simulink model "Sim_localization_template"  (R2024b)
settings: Solver=VariableStepAuto  StartTime=0.0  StopTime=80  MaxStep=0.001  RelTol=1e-3
undefined symbols (not defined in the file or in its folder): D, d, d_actual, P_INIT_EKF, PHI_INIT, prob_gps_loss, Q_INIT, Q_INIT_LOC, r, R_2, R_3, R_4, R_5, r_actual, T_s, Ta, Tc, Z_INIT_EKF
settings Model: Creator=alberto  LastModifiedBy=Riccardo
settings RTWCC: GPUComputeCapability=3.5

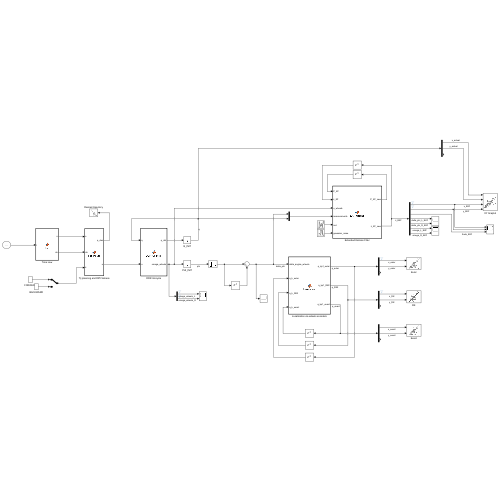
[thumbnail: Simulink's stored preview of the top-level diagram]
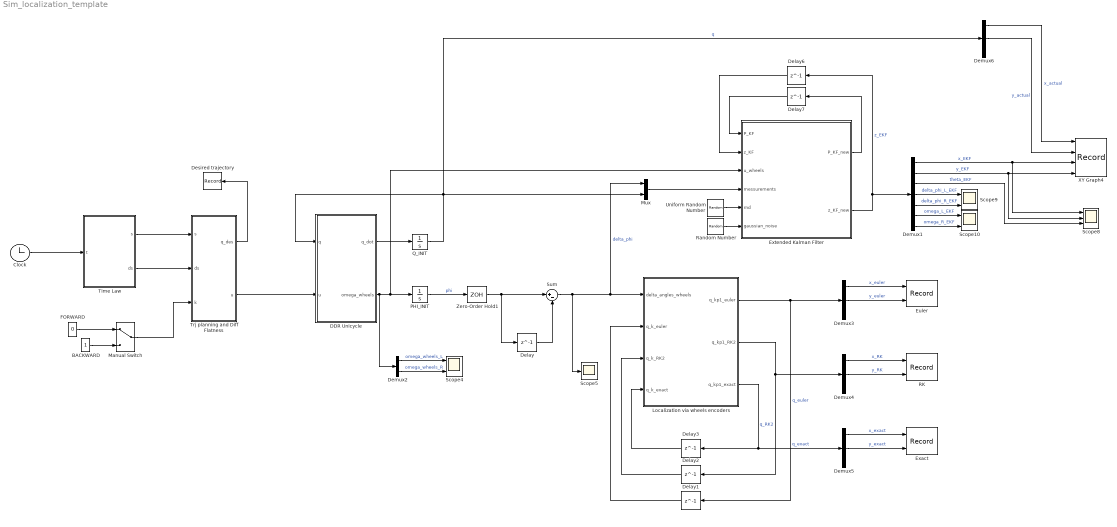
== system Sim_localization_template ==
  BACKWARD : Constant
  Clock : Clock
  DDR Unicycle : MATLAB Function  TreatAsAtomicUnit=on
  Delay : Delay  DelayLength=1  InitialCondition=[0;0]  SampleTime=T_s
  Delay1 : Delay  DelayLength=1  InitialCondition=Q_INIT_LOC
  Delay2 : Delay  DelayLength=1  InitialCondition=Q_INIT_LOC
  Delay3 : Delay  DelayLength=1  InitialCondition=Q_INIT_LOC
  Delay6 : Delay  DelayLength=1  InitialCondition=Z_INIT_EKF  SampleTime=T_s
  Delay7 : Delay  DelayLength=1  InitialCondition=P_INIT_EKF  SampleTime=T_s
  Demux1 : Demux  Outputs=7
  Demux2 : Demux  Outputs=2
  Demux{3..6} (4 alike) : Demux  Outputs=3
  Desired trajectory : Record  FileSettingsInternal="{\"entries\":[{\"content\":{\"excelSettings\":{\"content\":{},\"type\":\"Streamout.ExcelSettings\"}},\"type\":\"Streamout.FileSettingStorage\",\"uuid\":\"\"}],\"packageUris\":[\"http:\\/\\/schema.mathworks.com\\/mf0\\/streamout_blocks\\/R2020a\"],\"version\":\"1.0\"}"  Layout=[1 1]  SignalsInternal="{\"entries\":[{\"content\":{\"signals\":[{\"content\":{\"blockPath\":[],\"dimensions\":[3,1],\"domain\":\"\",\"hasChildren\":true,\"lineColor\":\"#0072bd\",\"lineWidth\":2,\"port\":1,\"sid\":[\"\"],\"signalID\":1,\"signalName\":\"Trj planning and Diff Flatness:1\"},\"type\":\"RecordBlkView.Signal\",\"uuid\":\"\"},{\"content\":{\"blockPath\":[],\"channel\":[1,1],\"dimensions\":[3,1],\"domain\":\"\",\"lineColor\":\"#b746ff\",\"lineWidth\":2,\"parentID\":1,\"plots\":[ 1 ],\"port\":1,\"sid\":[\"\"],\"signalID\":2,\"signalName\":\"Trj planning and Diff Flatness:1\"},\"type\":\"RecordBlkView.Signal\",\"uuid\":\"\"},{\"content\":{\"blockPath\":[],\"channel\":[2,1],\"dimensions\":[3,1],\"domain\":\"\",\"lineColor\":\"#64d413\",\"lineWidth\":2,\"parentID\":1,\"plots\":[ 1 ],\"port\":1,\"sid\":[\"\"],\"signalID\":3,\"signalName\":\"Trj planning and Diff Flatness:1\"},\"type\":\"RecordBlkView.Signal\",\"uuid\":\"\"},{\"content\":{\"blockPath\":[],\"channel\":[3,1],\"dimensions\":[3,1],\"domain\":\"\",\"lineColor\":\"#ff13a6\",\"lineWidth\":2,\"parentID\":1,\"port\":1,\"sid\":[\"\"],\"signalID\":4,\"signalName\":\"Trj planning and Diff Flatness:1\"},\"type\":\"RecordBlkView.Signal\",\"uuid\":\"\"}]},\"type\":\"RecordBlkView.InputSignals\",\"uuid\":\"\"}],\"packageUris\":[\"http:\\/\\/schema.mathworks.com\\/mf0\\/streamout_blocks\\/R2020a\"],\"version\":\"1.0\"}"  VisualizationBindings="{\"xyplotplugin\":{\"info\":[{\"series\":[{\"bindingParametersList\":[{\"parameter\":\"X-Axis\",\"signalID\":2,\"signalName\":\"Trj planning and Diff Flatness:1(1,1)\"},{\"parameter\":\"Y-Axis\",\"signalID\":3,\"signalName\":\"Trj planning and Diff Flatness:1(2,1)\"}],\"seriesID\":0}],\"subplotID\":1}]}}"  CompatibilityTag=XY
  Euler : Record  FileSettingsInternal="{\"entries\":[{\"content\":{\"excelSettings\":{\"content\":{},\"type\":\"Streamout.ExcelSettings\"}},\"type\":\"Streamout.FileSettingStorage\",\"uuid\":\"\"}],\"packageUris\":[\"http:\\/\\/schema.mathworks.com\\/mf0\\/streamout_blocks\\/R2020a\"],\"version\":\"1.0\"}"  Layout=[1 1]  SignalsInternal="{\"entries\":[{\"content\":{\"signals\":[{\"content\":{\"blockPath\":[],\"dimensions\":[1,1],\"domain\":\"\",\"lineColor\":\"#edb120\",\"lineWidth\":2,\"plots\":[ 1 ],\"port\":1,\"sid\":[\"\"],\"signalID\":1,\"signalName\":\"x_euler\"},\"type\":\"RecordBlkView.Signal\",\"uuid\":\"\"},{\"content\":{\"blockPath\":[],\"dimensions\":[1,1],\"domain\":\"\",\"lineColor\":\"#b746ff\",\"lineWidth\":2,\"plots\":[ 1 ],\"port\":2,\"sid\":[\"\"],\"signalID\":2,\"signalName\":\"y_euler\"},\"type\":\"RecordBlkView.Signal\",\"uuid\":\"\"}]},\"type\":\"RecordBlkView.InputSignals\",\"uuid\":\"\"}],\"packageUris\":[\"http:\\/\\/schema.mathworks.com\\/mf0\\/streamout_blocks\\/R2020a\"],\"version\":\"1.0\"}"  VisualizationBindings="{\"xyplotplugin\":{\"info\":[{\"series\":[{\"bindingParametersList\":[{\"parameter\":\"X-Axis\",\"signalID\":1,\"signalName\":\"x_euler\"},{\"parameter\":\"Y-Axis\",\"signalID\":2,\"signalName\":\"y_euler\"}],\"seriesID\":0}],\"subplotID\":1}]}}"  CompatibilityTag=XY
  Exact : Record  FileSettingsInternal="{\"entries\":[{\"content\":{\"excelSettings\":{\"content\":{},\"type\":\"Streamout.ExcelSettings\"}},\"type\":\"Streamout.FileSettingStorage\",\"uuid\":\"\"}],\"packageUris\":[\"http:\\/\\/schema.mathworks.com\\/mf0\\/streamout_blocks\\/R2020a\"],\"version\":\"1.0\"}"  Layout=[1 1]  SignalsInternal="{\"entries\":[{\"content\":{\"signals\":[{\"content\":{\"blockPath\":[],\"dimensions\":[1,1],\"domain\":\"\",\"lineColor\":\"#ff6929\",\"lineWidth\":2,\"plots\":[ 1 ],\"port\":1,\"sid\":[\"\"],\"signalID\":1,\"signalName\":\"x_exact\"},\"type\":\"RecordBlkView.Signal\",\"uuid\":\"\"},{\"content\":{\"blockPath\":[],\"dimensions\":[1,1],\"domain\":\"\",\"lineColor\":\"#b746ff\",\"lineWidth\":2,\"plots\":[ 1 ],\"port\":2,\"sid\":[\"\"],\"signalID\":2,\"signalName\":\"y_exact\"},\"type\":\"RecordBlkView.Signal\",\"uuid\":\"\"}]},\"type\":\"RecordBlkView.InputSignals\",\"uuid\":\"\"}],\"packageUris\":[\"http:\\/\\/schema.mathworks.com\\/mf0\\/streamout_blocks\\/R2020a\"],\"version\":\"1.0\"}"  VisualizationBindings="{\"xyplotplugin\":{\"info\":[{\"series\":[{\"bindingParametersList\":[{\"parameter\":\"X-Axis\",\"signalID\":1,\"signalName\":\"x_exact\"},{\"parameter\":\"Y-Axis\",\"signalID\":2,\"signalName\":\"y_exact\"}],\"seriesID\":0}],\"subplotID\":1}]}}"  CompatibilityTag=XY
  Extended Kalman Filter : MATLAB Function  TreatAsAtomicUnit=on
  FORWARD : Constant  Value=0
  Localization via wheels encoders : MATLAB Function  TreatAsAtomicUnit=on
  Manual Switch : ManualSwitch
  Mux : Mux  Inputs=2
  PHI_INIT : Integrator  InitialCondition=PHI_INIT
  Q_INIT : Integrator  InitialCondition=Q_INIT
  RK : Record  FileSettingsInternal="{\"entries\":[{\"content\":{\"excelSettings\":{\"content\":{},\"type\":\"Streamout.ExcelSettings\"}},\"type\":\"Streamout.FileSettingStorage\",\"uuid\":\"\"}],\"packageUris\":[\"http:\\/\\/schema.mathworks.com\\/mf0\\/streamout_blocks\\/R2020a\"],\"version\":\"1.0\"}"  Layout=[1 1]  SignalsInternal="{\"entries\":[{\"content\":{\"signals\":[{\"content\":{\"blockPath\":[],\"dimensions\":[1,1],\"domain\":\"\",\"lineColor\":\"#ff6929\",\"lineWidth\":2,\"plots\":[ 1 ],\"port\":1,\"sid\":[\"\"],\"signalID\":1,\"signalName\":\"x_RK\"},\"type\":\"RecordBlkView.Signal\",\"uuid\":\"\"},{\"content\":{\"blockPath\":[],\"dimensions\":[1,1],\"domain\":\"\",\"lineColor\":\"#b746ff\",\"lineWidth\":2,\"plots\":[ 1 ],\"port\":2,\"sid\":[\"\"],\"signalID\":2,\"signalName\":\"y_RK\"},\"type\":\"RecordBlkView.Signal\",\"uuid\":\"\"}]},\"type\":\"RecordBlkView.InputSignals\",\"uuid\":\"\"}],\"packageUris\":[\"http:\\/\\/schema.mathworks.com\\/mf0\\/streamout_blocks\\/R2020a\"],\"version\":\"1.0\"}"  VisualizationBindings="{\"xyplotplugin\":{\"info\":[{\"series\":[{\"bindingParametersList\":[{\"parameter\":\"X-Axis\",\"signalID\":1,\"signalName\":\"x_RK\"},{\"parameter\":\"Y-Axis\",\"signalID\":2,\"signalName\":\"y_RK\"}],\"seriesID\":0}],\"subplotID\":1}]}}"  CompatibilityTag=XY
  Random Number : RandomNumber  Variance=0.0001  SampleTime=T_s
  Scope10 : Scope  NumInputPorts=2
  Scope4 : Scope  NumInputPorts=2
  Scope5 : Scope
  Scope8 : Scope  NumInputPorts=3
  Scope9 : Scope  NumInputPorts=2
  Sum : Sum  Inputs=|+-
  Time Law : MATLAB Function  TreatAsAtomicUnit=on
  Trj planning and Diff Flatness : MATLAB Function  TreatAsAtomicUnit=on
  Uniform Random Number : UniformRandomNumber  Minimum=0  SampleTime=T_s
  XY Graph4 : Record  FileSettingsInternal="{\"entries\":[{\"content\":{\"excelSettings\":{\"content\":{},\"type\":\"Streamout.ExcelSettings\"}},\"type\":\"Streamout.FileSettingStorage\",\"uuid\":\"\"}],\"packageUris\":[\"http:\\/\\/schema.mathworks.com\\/mf0\\/streamout_blocks\\/R2020a\"],\"version\":\"1.0\"}"  Layout=[1 1]  SignalsInternal="{\"entries\":[{\"content\":{\"signals\":[{\"content\":{\"blockPath\":[],\"dimensions\":[1,1],\"domain\":\"\",\"lineColor\":\"#77ac30\",\"lineWidth\":2,\"plots\":[ 1 ],\"port\":1,\"sid\":[\"\"],\"signalID\":1,\"signalName\":\"x_actual\"},\"type\":\"RecordBlkView.Signal\",\"uuid\":\"\"},{\"content\":{\"blockPath\":[],\"dimensions\":[1,1],\"domain\":\"\",\"lineColor\":\"#4dbeee\",\"lineWidth\":2,\"plots\":[ 1 ],\"port\":2,\"sid\":[\"\"],\"signalID\":2,\"signalName\":\"y_actual\"},\"type\":\"RecordBlkView.Signal\",\"uuid\":\"\"},{\"content\":{\"blockPath\":[],\"dimensions\":[1,1],\"domain\":\"\",\"lineColor\":\"#a2142f\",\"lineWidth\":2,\"plots\":[ 1 ],\"port\":3,\"sid\":[\"\"],\"signalID\":3,\"signalName\":\"x_EKF\"},\"type\":\"RecordBlkView.Signal\",\"uuid\":\"\"},{\"content\":{\"blockPath\":[],\"dimensions\":[1,1],\"domain\":\"\",\"lineColor\":\"#139fff\",\"lineWidth\":2,\"plots\":[ 1 ],\"port\":4,\"sid\":[\"\"],\"signalID\":4,\"signalName\":\"y_EKF\"},\"type\":\"RecordBlkView.Signal\",\"uuid\":\"\"}]},\"type\":\"RecordBlkView.InputSignals\",\"uuid\":\"\"}],\"packageUris\":[\"http:\\/\\/schema.mathworks.com\\/mf0\\/streamout_blocks\\/R2020a\"],\"version\":\"1.0\"}"  VisualizationBindings="{\"xyplotplugin\":{\"info\":[{\"series\":[{\"bindingParametersList\":[{\"parameter\":\"X-Axis\",\"signalID\":1,\"signalName\":\"x_actual\"},{\"parameter\":\"Y-Axis\",\"signalID\":2,\"signalName\":\"y_actual\"}],\"seriesID\":0},{\"bindingParametersList\":[{\"parameter\":\"X-Axis\",\"signalID\":3,\"signalName\":\"x_EKF\"},{\"parameter\":\"Y-Axis\",\"signalID\":4,\"signalName\":\"y_EKF\"}],\"seriesID\":1}],\"subplotID\":1}]}}"  CompatibilityTag=XY
  Zero-Order Hold1 : ZeroOrderHold  SampleTime=T_s
  wires:
  Trj planning and Diff Flatness/2(u) -> DDR Unicycle/2(u)
  Zero-Order Hold1/1 -> Sum/1, Delay/1
  Delay/1 -> Sum/2
  Delay1/1 -> Localization via wheels encoders/2(q_k_euler)
  Sum/1 -> Mux/1, Localization via wheels encoders/1(delta_angles_wheels), Scope5/1  "delta_phi"
  Localization via wheels encoders/1(q_kp1_euler) -> Demux3/1, Delay1/1  "q_euler"
  Q_INIT/1 -> DDR Unicycle/1(q), Demux6/1, Mux/2  "q"
  Delay3/1 -> Localization via wheels encoders/4(q_k_exact)
  Delay2/1 -> Localization via wheels encoders/3(q_k_RK2)
  Localization via wheels encoders/2(q_kp1_RK2) -> Demux4/1, Delay2/1  "q_RK2"
  Time Law/1(s) -> Trj planning and Diff Flatness/1(s)
  Time Law/2(ds) -> Trj planning and Diff Flatness/2(ds)
  DDR Unicycle/1(q_dot) -> Q_INIT/1
  Trj planning and Diff Flatness/1(q_des) -> Desired trajectory/1
  DDR Unicycle/2(omega_wheels) -> Demux2/1, Extended Kalman Filter/3(u_wheels), PHI_INIT/1
  PHI_INIT/1 -> Zero-Order Hold1/1  "phi"
  Demux6/2 -> XY Graph4/2  "y_actual"
  Demux6/1 -> XY Graph4/1  "x_actual"
  Clock/1 -> Time Law/1(t)
  Demux3/1 -> Euler/1  "x_euler"
  Demux3/2 -> Euler/2  "y_euler"
  Extended Kalman Filter/1(P_KF_new) -> Delay7/1
  Extended Kalman Filter/2(z_KF_new) -> Demux1/1, Delay6/1  "z_EKF"
  Delay7/1 -> Extended Kalman Filter/1(P_KF)
  Delay6/1 -> Extended Kalman Filter/2(z_KF)
  Demux1/1 -> Scope8/1, XY Graph4/3  "x_EKF"
  Demux1/2 -> Scope8/2, XY Graph4/4  "y_EKF"
  Demux1/3 -> Scope8/3  "theta_EKF"
  Demux1/4 -> Scope9/1  "delta_phi_L_EKF"
  Demux1/5 -> Scope9/2  "delta_phi_R_EKF"
  Demux1/6 -> Scope10/1  "omega_L_EKF"
  Demux1/7 -> Scope10/2  "omega_R_EKF"
  Localization via wheels encoders/3(q_kp1_exact) -> Delay3/1, Demux5/1  "q_exact"
  Demux2/1 -> Scope4/1  "omega_wheels_L"
  Demux2/2 -> Scope4/2  "omega_wheels_R"
  Mux/1 -> Extended Kalman Filter/4(messurements)
  Uniform Random Number/1 -> Extended Kalman Filter/5(rnd)
  Random Number/1 -> Extended Kalman Filter/6(gaussian_noise)
  FORWARD/1 -> Manual Switch/1
  BACKWARD/1 -> Manual Switch/2
  Manual Switch/1 -> Trj planning and Diff Flatness/3(k)
  Demux4/2 -> RK/2  "y_RK"
  Demux4/1 -> RK/1  "x_RK"
  Demux5/2 -> Exact/2  "y_exact"
  Demux5/1 -> Exact/1  "x_exact"

== matlab function Sim_localization_template/Time Law ==
  data: t input; s output; ds output; Ta parameter; Tc parameter
function [s, ds] = fcn(t, Ta, Tc)
    
    v_c = 1/(Ta+Tc);
    a = v_c/Ta;

    if(t>=0 && t<Ta)
        s = (a*t^2)/2;
        ds = a*t;
    elseif(t>=Ta && t<Tc+Ta)
        s = a*Ta^2/2 + v_c*(t-Ta);
        ds = v_c;
    elseif(t>=(Ta+Tc) && t<(Tc+2*Ta))
        s = (a*Ta^2)/2 + v_c*(t-Ta-Tc) + v_c*Tc - (a*(t-Ta-Tc)^2)/2;
        ds = v_c - a*(t-Ta-Tc);
    else
        s = 1;
        ds = 0;
    end
end

== matlab function Sim_localization_template/DDR Unicycle ==
  data: q input; u input; q_dot output; omega_wheels output; d_actual parameter; r_actual parameter
function [q_dot,  omega_wheels]  = DDR_Unicycle(q, u, d_actual, r_actual)

omega_wheels = [u(1)/r_actual - d_actual*u(2)/(2*r_actual);
                u(1)/r_actual + d_actual*u(2)/(2*r_actual)];

q_dot = [cos(q(3))*u(1);
         sin(q(3))*u(1);
         u(2)];
end

== matlab function Sim_localization_template/Trj planning and Diff Flatness ==
  data: q_des output; s input; u output; ds input; k input
function [q_des, u] = get_inputs(s, ds, k)
    
    R = 0.5;            % radius for the 8-shaped trj
    omega_trj = 2*pi;   % trajectory completes one full cycle (2pi) per unit of s

    x_s = R*sin(2*omega_trj*s);
    y_s = R*sin(omega_trj*s);

    x_prime = R*2*omega_trj*cos(2*omega_trj*s);
    y_prime = R*omega_trj*cos(omega_trj*s);

    x_dotdot = -R*((2*omega_trj)^2)*sin(2*omega_trj*s);
    y_dotdot = -R*(omega_trj^2)*sin(omega_trj*s);

    if(k==0)
        v = sqrt((x_prime)^2+(y_prime)^2) * ds; %forward
    else
        v = -sqrt((x_prime)^2+(y_prime)^2) * ds; %backwards
    end

    w=(((x_prime)*(y_dotdot)-(y_prime)*(x_dotdot))/((x_prime)^2 + (y_prime)^2)) * ds;

    theta = (s*x_prime*y_dotdot)/(x_prime^2 + y_prime^2) - (s*y_prime*x_dotdot)/(x_prime^2 + y_prime^2);

    q_des = [x_s; y_s; theta];
    u = [v; w];
    
end

== matlab function Sim_localization_template/Localization via wheels encoders ==
  data: delta_angles_wheels input; q_k_euler input; q_k_RK2 input; q_k_exact input; r parameter; d parameter; q_kp1_euler output; T_s parameter; q_kp1_RK2 output; q_kp1_exact output
function [q_kp1_euler, q_kp1_RK2, q_kp1_exact] = localization(delta_angles_wheels, q_k_euler, q_k_RK2, q_k_exact, r, d, T_s)

v_k = r * (delta_angles_wheels(1) + delta_angles_wheels(2)) / (T_s * 2);
w_k = r * (delta_angles_wheels(2) - delta_angles_wheels(1)) / (T_s * d);

% Euler integration
x_kp1_euler     = q_k_euler(1) + T_s * v_k * cos(q_k_euler(3));
y_kp1_euler     = q_k_euler(2) + T_s * v_k * sin(q_k_euler(3));
theta_kp1_euler = q_k_euler(3) + T_s * w_k;
q_kp1_euler     = [x_kp1_euler; y_kp1_euler; theta_kp1_euler];

% Runge-Kutta 2
x_kp1_RK2       = q_k_RK2(1) + T_s * v_k * cos(q_k_RK2(3) + T_s * w_k / 2);
y_kp1_RK2       = q_k_RK2(2) + T_s * v_k * sin(q_k_RK2(3) + T_s * w_k / 2);
theta_kp1_RK2   = q_k_RK2(3) + T_s * w_k;
q_kp1_RK2       = [x_kp1_RK2; y_kp1_RK2; theta_kp1_RK2];

% Exact Integration
x_kp1_exact     = q_k_exact(1) + (v_k / w_k) * (sin(q_k_exact(3) + w_k*T_s) - sin(q_k_exact(3)));
y_kp1_exact     = q_k_exact(2) - (v_k / w_k) * (cos(q_k_exact(3) + w_k*T_s) - cos(q_k_exact(3)));
theta_kp1_exact = q_k_exact(3) + T_s * w_k;

% The problem with Exact integration fixed by switching strategy
if abs(delta_angles_wheels(2) - delta_angles_wheels(1)) <= 0.001
    q_kp1_exact = [x_kp1_RK2; y_kp1_RK2; theta_kp1_RK2];
else
    q_kp1_exact = [x_kp1_exact; y_kp1_exact; theta_kp1_exact];
end

end

== matlab function Sim_localization_template/Extended Kalman Filter ==
  data: P_KF input; P_KF_new output; z_KF input; z_KF_new output; u_wheels input; messurements input; D parameter; R_2 parameter; R_3 parameter; R_4 parameter; R_5 parameter; T_s parameter; r parameter; d parameter; prob_gps_loss parameter; rnd input; gaussian_noise input
function [P_KF_new, z_KF_new] = EKF_filtering(P_KF, z_KF, u_wheels, messurements, D, R_2, R_3, R_4, R_5 ,T_s, r, d, prob_gps_loss, rnd, gaussian_noise)

% z_KF = [x_EKF, y_EKF, theta_EKF, delta_phi_L_EKF, delta_phi_R_EKF, omega_L_EKF, omega_R_EKF]

v_k = r * (z_KF(6) + z_KF(7))/2;
w_k = r * (z_KF(7) - z_KF(6))/d;

theta_mean = z_KF(3) + (w_k * T_s)/2;

F_k = [1, 0, -T_s * v_k * sin(theta_mean), 0, 0, T_s * r * cos(theta_mean)/2 + (T_s)^2 * r * v_k * sin(theta_mean)/(2*d), T_s * r * cos(theta_mean)/2 - (T_s)^2 * r * v_k * sin(theta_mean)/(2*d);
    0, 1, T_s * v_k * cos(theta_mean), 0, 0, T_s * r * sin(theta_mean)/2 - (T_s)^2 * r * v_k * cos(theta_mean)/(2*d), T_s * r * sin(theta_mean)/2 + (T_s)^2 * r * v_k * cos(theta_mean)/(2*d);
    0, 0, 1, 0, 0, (-T_s*r)/d, (T_s*r)/d;
    0, 0, 0, 0, 0, T_s, 0;
    0, 0, 0, 0, 0, 0, T_s;
    0, 0, 0, 0, 0, 0, 0;
    0, 0, 0, 0, 0, 0, 0];

%% Prediction part

z_pred = [z_KF(1)+(T_s*r*(z_KF(6)+z_KF(7))/2)*cos(theta_mean + (T_s*r*(z_KF(6)+z_KF(7)))/(2*d));
    z_KF(2)+(T_s*r*(z_KF(6)+z_KF(7))/2)*sin(theta_mean + (T_s*r*(z_KF(7)-z_KF(6)))/(2*d));
    theta_mean + (T_s*r*(z_KF(7)-z_KF(6))/(2*d));
    T_s*z_KF(6);
    T_s*z_KF(7);
    u_wheels(1);
    u_wheels(2)];

P_pred = F_k * P_KF * F_k' + D;


%% Update

if(rnd<prob_gps_loss) 

    % Just encoders
    y_messurement = [messurements(1); messurements(2)];
    H = [0, 0, 0, 1, 0, 0, 0;
        0, 0, 0, 0, 1, 0, 0];

    e = y_messurement - H * z_pred;
    K = P_pred * H' /(H * P_pred * H' + R_2);

    z_KF_new = z_pred +  K * e;
    P_KF_new = P_pred - K * H * P_pred;

else 
    % GPS + Encoders
    y_messurement = [messurements(3)+gaussian_noise;messurements(4)+gaussian_noise;messurements(5)+gaussian_noise; messurements(1); messurements(2)];

    H = [1, 0, 0, 0, 0, 0, 0;
         0, 1, 0, 0, 0, 0, 0;
         0, 0, 1, 0, 0, 0, 0;
         0, 0, 0, 1, 0, 0, 0;
         0, 0, 0, 0, 1, 0, 0];

    e = y_messurement - H * z_pred;
    K = P_pred * H' /(H * P_pred * H' + R_5);

    z_KF_new = z_pred + K * e;
    P_KF_new = P_pred - K * H * P_pred;

end
